simulink model "tryout"  (R2023b)
settings: Solver=ode4  StartTime=0.0  StopTime=1  FixedStep=0.1  RelTol=1e-3
values from neighbouring files (symbols this model uses):
  M = M_a + M_rb    [EOM_input.m]    (also in Mechatronics (1).m; Mechatronics.m)
  tau = [tau_u;tau_v;tau_r]    [EOM_input.m]    (also in Mechatronics (1).m; Mechatronics.m)
  tau_e = [0; 0; 0]    [EOM_input.m]    (also in Mechatronics (1).m = 0; Mechatronics.m = [0 0 0])
libraries: matrix_library x2
settings Model: Creator=chris  LastModifiedBy=chris

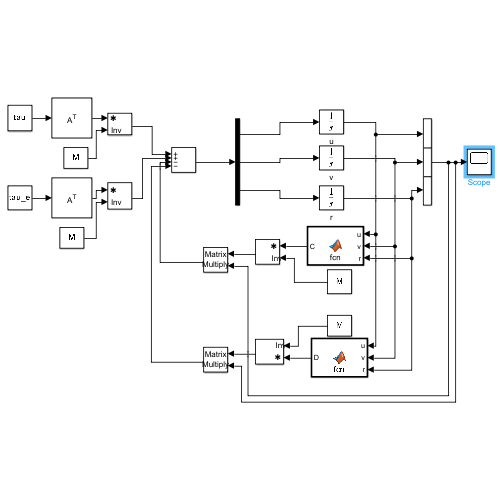
[thumbnail: Simulink's stored preview of the top-level diagram]
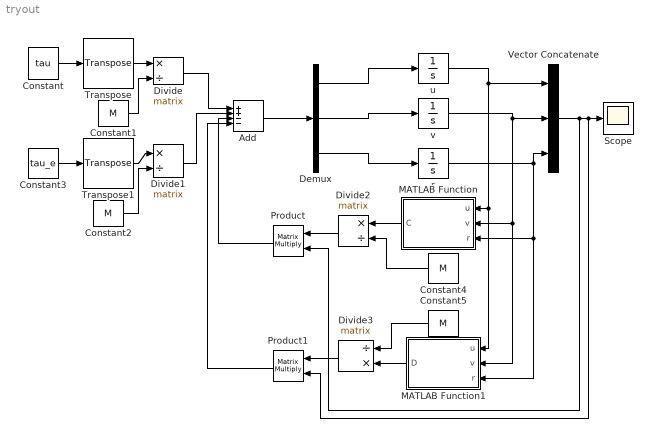
== system tryout ==
  Add : Sum  Inputs=++--
  Constant : Constant  Value=tau
  Constant{1..2,4..5} (4 alike) : Constant  Value=M
  Constant3 : Constant  Value=tau_e
  Demux : Demux  Outputs=3
  Divide : Product  Inputs=*/  Multiplication=Matrix(*)
  Divide1 : Product  Inputs=*/  Multiplication=Matrix(*)
  Divide2 : Product  Inputs=*/  Multiplication=Matrix(*)
  Divide3 : Product  Inputs=/*  Multiplication=Matrix(*)
  MATLAB Function : MATLAB Function  TreatAsAtomicUnit=on
  MATLAB Function1 : MATLAB Function  TreatAsAtomicUnit=on
  Product : Product  Multiplication=Matrix(*)
  Product1 : Product  Multiplication=Matrix(*)
  Scope : Scope
  Transpose : matrix_library/Transpose
  Transpose1 : matrix_library/Transpose
  Vector Concatenate : Concatenate  NumInputs=3
  r : Integrator
  u : Integrator
  v : Integrator
  wires:
  Constant/1 -> Transpose/1
  Constant1/1 -> Divide/2
  Constant3/1 -> Transpose1/1
  Divide/1 -> Add/1
  Divide1/1 -> Add/2
  Add/1 -> Demux/1
  Demux/1 -> u/1
  Demux/2 -> v/1
  Demux/3 -> r/1
  u/1 -> MATLAB Function1/1(u), MATLAB Function/1(u), Vector Concatenate/1
  v/1 -> Vector Concatenate/2, MATLAB Function1/2(v), MATLAB Function/2(v)
  r/1 -> Vector Concatenate/3, MATLAB Function/3(r), MATLAB Function1/3(r)
  Vector Concatenate/1 -> Product/2, Product1/2, Scope/1
  MATLAB Function/1(C) -> Divide2/1
  Divide2/1 -> Product/1
  Product/1 -> Add/3
  MATLAB Function1/1(D) -> Divide3/2
  Product1/1 -> Add/4
  Transpose/1 -> Divide/1
  Transpose1/1 -> Divide1/1
  Constant2/1 -> Divide1/2
  Constant5/1 -> Divide3/1
  Constant4/1 -> Divide2/2
  Divide3/1 -> Product1/1

== matlab function tryout/MATLAB Function ==
  data: u input; C output; v input; r input
function C = fcn(u, v, r)
x_g = 0; % body fixed reference system located at COG
y_g = 0;
m = 18; % Mass

C_rb = [0,0, -m*(x_g*r+v);
        0,0, -m*(y_g*r-u);
        m*(x_g*r + v), m*(y_g*r- u),0];

w = 0; % heave
p = 0; % roll
q = 0; % pitch

X_dotu = 1.2; % all of this given
X_dotv = 0;
X_dotw = 0;
X_dotp = 0;
X_dotq = 0;
X_dotr = 0;

Y_dotu = 0; 
Y_dotv = 66.1; 
Y_dotw = 0;
Y_dotp = 0;
Y_dotq = 0;
Y_dotr = 0;

a_1 = X_dotu*u + X_dotv*v +X_dotw*w + X_dotp*p + X_dotq*q +X_dotr*r;
a_2 = Y_dotu*u + Y_dotv*v +Y_dotw*w + Y_dotp*p + Y_dotq*q +Y_dotr*r;

C_a = [0,   0,   a_2;
       0,   0,  -a_1;
      -a_2, a_1,  0];

C = C_rb + C_a;

== matlab function tryout/MATLAB Function1 ==
  data: u input; D output; v input; r input
function D = fcn(u, v, r)
d_11 = 0.0069*u^3 - 0.1314*u^2 + 0.8842*u - 2.0431;  %X_drag
d_22 = 0.0289*v^3 - 0.5191*v^2 + 3.3058*v - 2.3601;  %Y_drag
c1 = 122.3;
c2 = 4.8;
L = 0.97;
d_33 = (1/80)*c1*r^3*L^4 + (1/12)*c2*r*L^2;

D = [d_11, 0,   0;
      0,  d_22, 0;
      0,   0,  d_33];
